simulink model "NL_cartmodel"  (R2019b)
settings: Solver=ode4  StartTime=0.0  StopTime=stoptime  FixedStep=h  RelTol=1e-3
values from neighbouring files (symbols this model uses):
  A = Ab    [mainfile_solution.m]
  b = 1    [mainfile_solution.m]
  B = Bb    [mainfile_solution.m]
  C = Cb    [mainfile_solution.m]
  controller_enabled = 1    [mainfile_solution.m]
  g = 9.81    [mainfile_solution.m]
  K = place(A,B,p)    [mainfile_solution.m]
  l = 0.2    [mainfile_solution.m]
  L = place(A',C',p)'    [mainfile_solution.m]
  m = 0.15    [mainfile_solution.m]
  Mc = 0.4    [mainfile_solution.m]
  use_state_estimates = 1    [mainfile_solution.m]
  x0 = x0b    [mainfile_solution.m]
  x_bar = xb_bar    [mainfile_solution.m]
settings Model: Creator=n9182250  LastModifiedBy=n9182250
settings DebuggingCC: ArithmeticOperatorsInVariantConditions=warning
settings SFSimCC: CustomCodeUndefinedFunction=UseInterfaceOnly

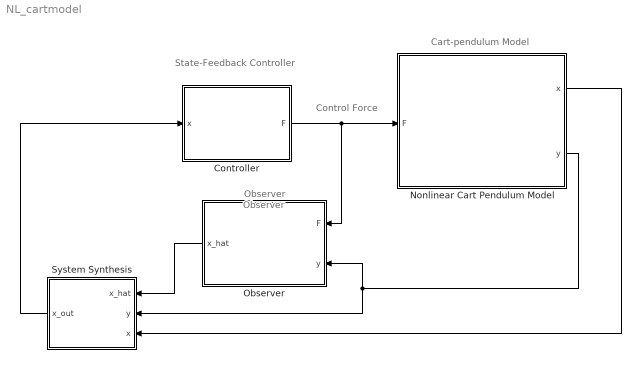
== system NL_cartmodel ==
  note: Control Force
  note: Cart-pendulum Model
  note: State-Feedback Controller
  note: Observer
  note: Observer
  Controller : Subsystem
  Nonlinear Cart Pendulum Model : Subsystem
  Observer : Subsystem
  System Synthesis : Subsystem
  wires:
  Nonlinear Cart Pendulum Model/2(y) -> System Synthesis/2(y), Observer/2(y)
  Controller/1(F) -> Observer/1(F), Nonlinear Cart Pendulum Model/1(F)
  Nonlinear Cart Pendulum Model/1(x) -> System Synthesis/3(x)
  Observer/1(x_hat) -> System Synthesis/1(x_hat)
  System Synthesis/1(x_out) -> Controller/1(x)

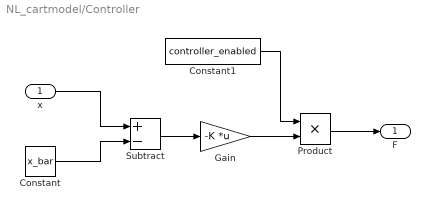
== system NL_cartmodel/Controller ==
  x : Inport
  Constant : Constant  Value=x_bar
  Constant1 : Constant  Value=controller_enabled
  Gain : Gain  Gain=-K  Multiplication=Matrix(K*u)
  Product : Product
  Subtract : Sum  Inputs=+-
  F : Outport
  wires:
  x/1 -> Subtract/1
  Constant/1 -> Subtract/2
  Subtract/1 -> Gain/1
  Constant1/1 -> Product/1
  Gain/1 -> Product/2
  Product/1 -> F/1

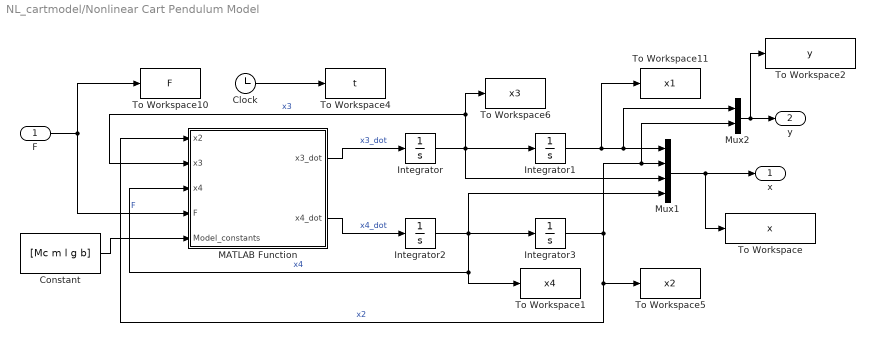
== system NL_cartmodel/Nonlinear Cart Pendulum Model ==
  F : Inport
  Clock : Clock
  Constant : Constant  Value=[Mc m l g b]
  Integrator : Integrator  InitialCondition=x0(3)
  Integrator1 : Integrator  InitialCondition=x0(1)
  Integrator2 : Integrator  InitialCondition=x0(4)
  Integrator3 : Integrator  InitialCondition=x0(2)
  MATLAB Function : MATLAB Function  TreatAsAtomicUnit=on
  Mux1 : Mux
  Mux2 : Mux  Inputs=2
  To Workspace : ToWorkspace  VariableName=x  SampleTime=-1
  To Workspace1 : ToWorkspace  VariableName=x4  SampleTime=-1
  To Workspace10 : ToWorkspace  VariableName=F  SampleTime=-1
  To Workspace11 : ToWorkspace  VariableName=x1  SampleTime=-1
  To Workspace2 : ToWorkspace  VariableName=y  SampleTime=-1
  To Workspace4 : ToWorkspace  VariableName=t  SampleTime=-1
  To Workspace5 : ToWorkspace  VariableName=x2  SampleTime=-1
  To Workspace6 : ToWorkspace  VariableName=x3  SampleTime=-1
  x : Outport  VectorParamsAs1DForOutWhenUnconnected=off
  y : Outport  Port=2  VectorParamsAs1DForOutWhenUnconnected=off
  wires:
  Mux1/1 -> x/1, To Workspace/1
  MATLAB Function/1(x3_dot) -> Integrator/1  "x3_dot"
  Integrator3/1 -> MATLAB Function/1(x2), To Workspace5/1, Mux2/2, Mux1/2  "x2"
  Integrator1/1 -> Mux2/1, Mux1/1, To Workspace11/1
  MATLAB Function/2(x4_dot) -> Integrator2/1  "x4_dot"
  Integrator/1 -> To Workspace6/1, MATLAB Function/2(x3), Mux1/3, Integrator1/1  "x3"
  F/1 -> MATLAB Function/4(F), To Workspace10/1  "F"
  Integrator2/1 -> MATLAB Function/3(x4), To Workspace1/1, Mux1/4, Integrator3/1  "x4"
  Clock/1 -> To Workspace4/1
  Mux2/1 -> y/1, To Workspace2/1
  Constant/1 -> MATLAB Function/5(Model_constants)

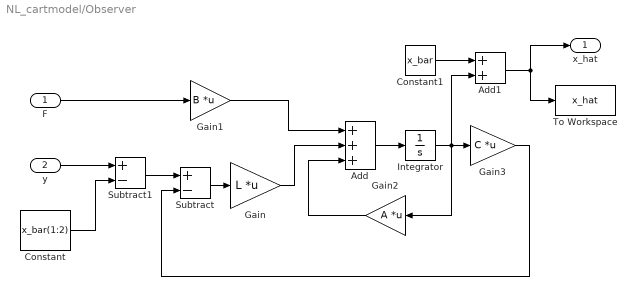
== system NL_cartmodel/Observer ==
  F : Inport
  y : Inport  Port=2
  Add : Sum  Inputs=+++
  Add1 : Sum
  Constant : Constant  Value=x_bar(1:2)
  Constant1 : Constant  Value=x_bar
  Gain : Gain  Gain=L  Multiplication=Matrix(K*u)
  Gain1 : Gain  Gain=B  Multiplication=Matrix(K*u)
  Gain2 : Gain  Gain=A  Multiplication=Matrix(K*u)
  Gain3 : Gain  Gain=C  Multiplication=Matrix(K*u)
  Integrator : Integrator
  Subtract : Sum  Inputs=+-
  Subtract1 : Sum  Inputs=+-
  To Workspace : ToWorkspace  VariableName=x_hat  SampleTime=-1
  x_hat : Outport  VectorParamsAs1DForOutWhenUnconnected=off
  wires:
  Subtract/1 -> Gain/1
  F/1 -> Gain1/1
  Gain1/1 -> Add/1
  Gain/1 -> Add/2
  Add/1 -> Integrator/1
  Gain2/1 -> Add/3
  Integrator/1 -> Add1/2, Gain2/1, Gain3/1
  Gain3/1 -> Subtract/2
  y/1 -> Subtract1/1
  Subtract1/1 -> Subtract/1
  Constant/1 -> Subtract1/2
  Constant1/1 -> Add1/1
  Add1/1 -> x_hat/1, To Workspace/1

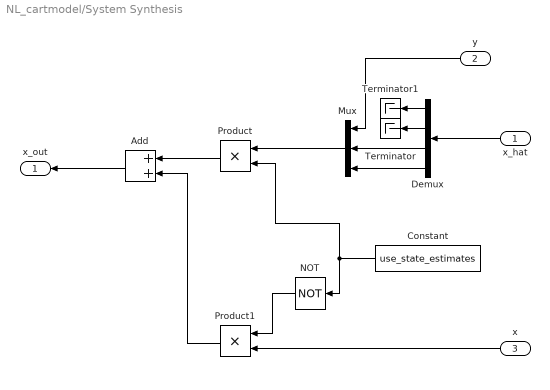
== system NL_cartmodel/System Synthesis ==
  x_hat : Inport
  y : Inport  Port=2
  x : Inport  Port=3
  Add : Sum
  Constant : Constant  Value=use_state_estimates
  Demux : Demux
  Mux : Mux  Inputs=3
  NOT : Logic  Operator=NOT  IconShape=distinctive  AllPortsSameDT=off  OutDataTypeStr=boolean
  Product : Product
  Product1 : Product
  Terminator : Terminator
  Terminator1 : Terminator
  x_out : Outport
  wires:
  Demux/1 -> Terminator1/1
  Demux/2 -> Terminator/1
  Demux/3 -> Mux/2
  Demux/4 -> Mux/3
  y/1 -> Mux/1
  x_hat/1 -> Demux/1
  Mux/1 -> Product/1
  Constant/1 -> Product/2, NOT/1
  x/1 -> Product1/2
  NOT/1 -> Product1/1
  Add/1 -> x_out/1
  Product/1 -> Add/1
  Product1/1 -> Add/2

== matlab function NL_cartmodel/Nonlinear Cart Pendulum Model/MATLAB Function ==
  data: x3_dot output; x2 input; x3 input; x4 input; F input; x4_dot output; Model_constants input
function [x3_dot,x4_dot] = NonLinearEquations(x2,x3,x4,F,Model_constants)

%Get Model Constants:
Mc = Model_constants(1);
m = Model_constants(2);
l = Model_constants(3);
g = Model_constants(4);
b = Model_constants(5);

%x3_dot equation
x3_dot = (x4^2*l*m*sin(x2)-g*m*sin(x2)*cos(x2)+F-b*x3)...
    /(Mc+m-m*(cos(x2))^2);

%x4_dot equation
x4_dot = (-l*m*sin(x2)*cos(x2)*x4^2+g*(Mc+m)*sin(x2)...
    -cos(x2)*F+b*x3*cos(x2))/(l*(Mc+m-m*(cos(x2))^2));
